simulink model "gdnn_lm_rtrl"  (R2023a)
settings: Solver=ode5  StartTime=0.0  StopTime=train_length  FixedStep=T_sim  RelTol=1e-3  EnableMultiTasking=on
values from neighbouring files (symbols this model uses):
  aa = (((m*l)^2)*g)/AA    (= 0.275046740282)    [init_model.m]
  bb = zeros(1, numoflayers)    [ini_gdnn.m]    (also in init_model.m = 0.588785047389)
  bs = zeros(1, numoflayers)    [ini_gdnn.m]
  cc = (b*m*l)/AA    (= 4.42542074273e-05)    [init_model.m]
  D_max = max(max(max(max(idel))),max(max(max(ldel))))    [ini_gdnn.m]
  dd = (m*g*l*(M+m))/AA    (= 6.05102828621)    [init_model.m]
  DI_vec = [DI_vec DI(i,:)]    [ini_gdnn.m]
  DIB_vec = [DIB_vec DIB(i,:)]    [ini_gdnn.m]
  dimax = max(dimax)    [ini_gdnn.m]
  DIS_vec = [DIS_vec DIS(i,:)]    [ini_gdnn.m]
  DL_vec = [DL_vec DL(i,:)]    [ini_gdnn.m]
  DLB_vec = [DLB_vec DLB(i,:)]    [ini_gdnn.m]
  dlmax = max(dlmax)    [ini_gdnn.m]
  DLS_vec = [DLS_vec DLS(i,:)]    [ini_gdnn.m]
  E_LW_U = zeros(1,numoflayers^2)    [ini_gdnn.m]
  ee = (m*l*c)/AA    (= 0.353271042564)    [init_model.m]
  ff = ((M+m)*b)/AA    (= 0.0009735925634)    [init_model.m]
  I = zeros(1,numoflayers*numofinputs)    [ini_gdnn.m]    (also in init_model.m = 0.05833333)
  idelb_vec = 0    [ini_gdnn.m]
  idels_vec = 0    [ini_gdnn.m]
  Lb = zeros(1,numoflayers^2)    [ini_gdnn.m]
  ldelb_vec = 0    [ini_gdnn.m]
  ldels_vec = 0    [ini_gdnn.m]
  Lf = zeros(1,numoflayers^2)    [ini_gdnn.m]
  mm = (I +m*(l^2))/AA    (= 0.9345794403)    [init_model.m]
  net_params = [Q, mue, theta, T, L, D_max, numoflayers, numofinputs, max(S), sum(R), S_out, S_target, print_weights, min_weights, prune_interval, train_length, prune_maxerr_OBS, prune_maxerr_exact]    [ini_gdnn.m]
  nn = (m*l)/AA    (= 0.56074768661)    [init_model.m]
  oo = (2*l*(M+m))/AA    (= 12.3364491054)    [init_model.m]
  Q = 500    [ini_gdnn.m]
  T = 0.01    [ini_gdnn.m]
  thetastart = pi    (= 3.14159265359)    [init_model.m]
  thetastartdelta = 10*(pi/180)    (= 0.174532925199)    [init_model.m]
  U = U_target    [ini_gdnn.m]
  U_out = zeros(1, numoflayers)    [ini_gdnn.m]
  U_target = zeros(1, numoflayers)    [ini_gdnn.m]
  W_alpha_ini = ones(1,L)    [ini_gdnn.m]
  W_ini = rand(1,L) - 0.5    [ini_gdnn.m]
  X = zeros(1,numoflayers)    [ini_gdnn.m]
  xstart = 0.0    (= 0)    [init_model.m]
  xstartdelta = 0.0    (= 0)    [init_model.m]
undefined symbols (not defined in the file or in its folder): idel_vec, ldel_vec, R, S
libraries: simulink x2, slpidlib x1
settings Model: Creator=endisch  LastModifiedBy=Wolfgang
settings SolverCC: AlgebraicLoopSolver=TrustRegion
settings DataIOCC: LimitDataPoints=on  SaveFormat=Array  SignalLoggingSaveFormat=ModelDataLogs  ReturnWorkspaceOutputs=off
settings OptimizationCC: InitFltsAndDblsToZero=on  LifeSpan=inf
settings DebuggingCC: SaveWithParameterizedLinksMsg=none  UnderspecifiedInitializationDetection=Classic  MergeDetectMultiDrivingBlocksExec=none  SignalResolutionControl=TryResolveAllWithWarning  SolverPrmCheckMsg=warning  MultiTaskDSMMsg=warning  MultiTaskCondExecSysMsg=none  FcnCallInpInsideContextMsg=warning  UnconnectedInputMsg=warning  UnconnectedOutputMsg=warning  UnconnectedLineMsg=warning  StateNameClashWarn=warning  SFUnexpectedBacktrackingDiag=warning  SFNoUnconditionalDefaultTransitionDiag=warning  SFExecutionAtInitializationDiag=none  ArithmeticOperatorsInVariantConditions=warning
settings HardwareCC: ProdBitPerPointer=32  ProdBitPerSizeT=32  ProdBitPerPtrDiffT=32  ProdLargestAtomicFloat=None  ProdIntDivRoundTo=Undefined  ProdEndianess=Unspecified  ProdWordSize=32  ProdHWDeviceType=32-bit Generic
settings ModelReferenceCC: EnableRefExpFcnMdlSchedulingChecks=on  PropagateSignalLabelsOutOfModel=off
settings SFSimCC: SimUseLocalCustomCode=off  CustomCodeUndefinedFunction=UseInterfaceOnly
settings RTWCC: RTWUseLocalCustomCode=off
settings CodeAppCC: StateflowObjectComments=on
settings GRTTargetCC: TargetFcnLib=ansi_tfl_tmw.mat  TargetLangStandard=C89/C90 (ANSI)  CombineOutputUpdateFcns=off  GRTInterface=on
settings ConfigComp: CovMetricSettings=dw  CovSaveCumulativeToWorkspaceVar=on  CovSaveSingleToWorkspaceVar=on  CovExternalEMLEnable=off

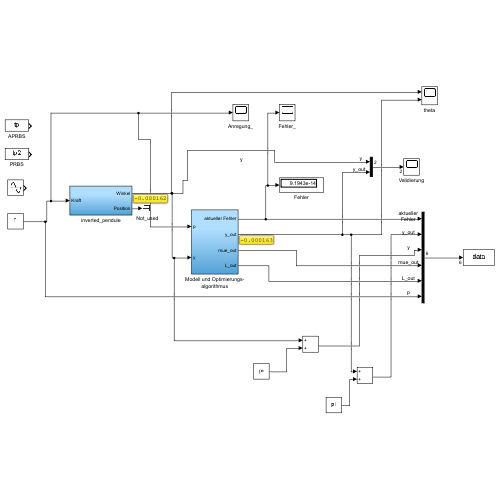
[thumbnail: Simulink's stored preview of the top-level diagram]
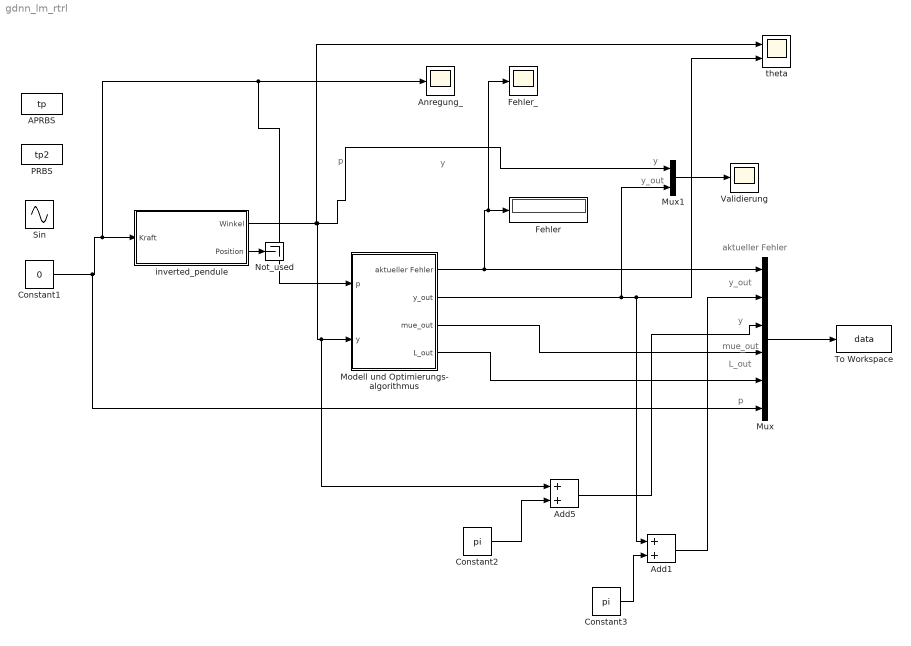
== system gdnn_lm_rtrl ==
  note: y_out
  note: y
  note: y
  note: p
  note: aktueller
      | Fehler
  note: y_out
  note: y
  note: mue_out
  note: L_out
  note: p
  APRBS : FromWorkspace  VariableName=tp  SampleTime=T  Interpolate=off  ZeroCross=off  OutputAfterFinalValue=Cyclic repetition
  Add1 : Sum
  Add5 : Sum
  Anregung_ : Scope
  Constant1 : Constant  Value=0
  Constant2 : Constant  Value=pi
  Constant3 : Constant  Value=pi
  Fehler : Display
      settings: Format=short_e
  "Fehler_ " : Scope
  Modell und Optimierungs- algorithmus : Subsystem
  Mux : Mux  Inputs=6
  Mux1 : Mux  Inputs=2
  Not_used : Terminator
  PRBS : FromWorkspace  VariableName=tp2  SampleTime=T  Interpolate=off  ZeroCross=off  OutputAfterFinalValue=Cyclic repetition
  Sin : Sin  Frequency=0.1  SampleTime=0
  To Workspace : ToWorkspace  VariableName=data  SaveFormat=Structure With Time  SampleTime=-1
  Validierung : Scope
  "inverted_pendule " : Subsystem  AncestorBlock=nichtlinearitaeten/Narendra Example 4
      settings: LibrarySourceBlock=|
      | nichtlinearitaeten/Narendra
      | Example 4
  theta : Scope  NumInputPorts=2
  wires:
  Mux/1 -> To Workspace/1
  "inverted_pendule "/1(Winkel) -> theta/1, Mux1/1, Add5/1, Modell und Optimierungs- algorithmus/2(y)
  Modell und Optimierungs- algorithmus/1(aktueller Fehler) -> "Fehler_ "/1, Fehler/1, Mux/1
  Modell und Optimierungs- algorithmus/3(mue_out) -> Mux/4
  Modell und Optimierungs- algorithmus/4(L_out) -> Mux/5
  Mux1/1 -> Validierung/1
  Modell und Optimierungs- algorithmus/2(y_out) -> Mux1/2, Add1/1, theta/2
  "inverted_pendule "/2(Position) -> Not_used/1
  Add5/1 -> Mux/3
  Constant2/1 -> Add5/2
  Add1/1 -> Mux/2
  Constant3/1 -> Add1/2
  Constant1/1 -> Mux/6, Modell und Optimierungs- algorithmus/1(p), Anregung_/1, "inverted_pendule "/1(Kraft)

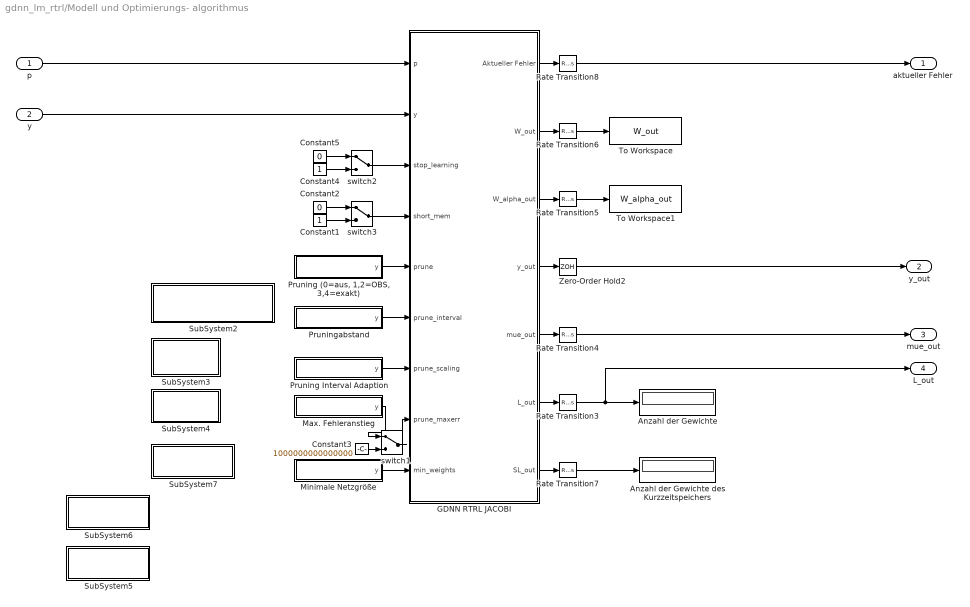
== system gdnn_lm_rtrl/Modell und Optimierungs- algorithmus ==
  p : Inport
  y : Inport  Port=2
  Anzahl der Gewichte : Display
  Anzahl der Gewichte des Kurzzeitspeichers : Display
  Constant1 : Constant
  Constant2 : Constant  Value=0
  Constant3 : Constant  Value=1000000000000000
  Constant4 : Constant
  Constant5 : Constant  Value=0
  GDNN RTRL JACOBI : Subsystem  TreatAsAtomicUnit=on  SystemSampleTime=T
  Max. Fehleranstieg : Subsystem  TreatAsAtomicUnit=on  SystemSampleTime=T  mask(Max. Error After Pruning-Step){number=10}
      mask prompts: number "Max. zulässig ist alter Fehler mal:"
      mask help: 0: Slider inaktiv, Wert wird aus der Ini-Datei (ini_gdnn.m) genommen
      mask Display: disp(sprintf('Fehleranstieg: %.1f',number));
  Minimale Netzgröße : Subsystem  TreatAsAtomicUnit=on  SystemSampleTime=T  mask(Minimum Number of Weights){number=1}
      mask prompts: number "Minimale Anzahl an Gewichte:"
      mask help: 0: Slider inaktiv, Wert wird aus der Ini-Datei (ini_gdnn.m) genommen
      mask Display: disp(sprintf('Gewichte: %i',number));
  "Pruning (0=aus, 1,2=OBS, 3,4=exakt)" : Subsystem  TreatAsAtomicUnit=on  SystemSampleTime=T  mask(Pruning Algorithms){number=0}
      mask prompts: number "Pruningverfahren:"
      mask help:
      | 0: aus
      | 1: OBS
      | 2: OBS, Berücksichtigung der Verzögerungsordnung
      | 3: exaktes Pruning
      | 4: exaktes Pruning, Berücksichtigung der Verzögerungsordnung
      mask TypeOptions number: 0 | 1 | 2 | 3 | 4
      mask Display: disp(sprintf('pruning %i',number-1));
  Pruning Interval Adaption : Subsystem  TreatAsAtomicUnit=on  SystemSampleTime=T  mask(Pruning Interval adaption){number=1}
      mask prompts: number "Skalierungsfaktor"
      mask help: 1.0: Pruning Interval wird nicht angepasst, Pruning Interval ist konstant
      mask Display: disp(sprintf('Scaling: %.1f',number));
  Pruningabstand : Subsystem  TreatAsAtomicUnit=on  SystemSampleTime=T  mask(Pruning Interval){number=100}
      mask prompts: number "Intervall (Abstand zweier Pruningschritte):"
      mask help: 0: Slider inaktiv, Wert wird aus der Ini-Datei (ini_gdnn.m) genommen
      mask Display: disp(sprintf('Intervall: %i',number));
  Rate Transition{3..8} (6 alike) : RateTransition  OutPortSampleTime=T
  SubSystem2 : Subsystem
      settings: OpenFcn=edit ini_gdnn.m gdnn_jacobi_rtrl.c forward_step.c get_jacobi_rtrl.c mem_alloc.c mem_free.c pruning_OBS.c w_conv.c transfer.c m_inv.c shift.c print_weights.c definitions.h;
      mask Display: disp('Load source files into editor\n(Double-Click)')
  SubSystem3 : Subsystem
      settings: OpenFcn="mex -v gdnn_jacobi_rtrl.c forward_step.c  get_jacobi_rtrl.c w_conv.c shift.c transfer.c m_inv.c pruning1_4.c mem_alloc.c mem_free.c print_weights.c"
      mask Display: disp('Mex files\n(Double-Click)')
  SubSystem4 : Subsystem
      settings: OpenFcn=clc
      mask Display: disp('Clear screen\n(Double-Click)')
  SubSystem5 : Subsystem
      settings: OpenFcn=|
      | net_params2 = net_params;
      | Q2=Q;
      | D_max2=D_max;
      | 
      | 
      | R2 = R;
      | S2 = S;
      | U2 = U;
      | X2 = X;
      | I2 = I;
      | Lf2 = Lf;
      | Lb2 = Lb;
      | E_LW_U2 = E_LW_U;
      | DI_vec2 = DI_vec;
      | DL_vec2 = DL_vec;
      | dimax2 = dimax;
      | dlmax2 = dlmax;
      | U_out2 = U_out;
      | U_target2 = U_target;
      | W_ini2 = W_out;
      | W_alpha_ini2 = W_alpha_out;
      | idel_vec2 = idel_vec;
      | ldel_vec2 = ldel_vec;
      | 
      | DIS_vec2=DIS_vec;
      | 
      | DLS_vec2=DLS_vec;
      | 
      | idels_vec2=idels_vec;
      | 
      | ldels_vec2=ldels_vec;
      | 
      | bs2=bs;
      | 
      | DIB_vec2=DIB_vec;
      | 
      | DLB_vec2=DLB_vec;
      | 
      | idelb_vec2=idelb_vec;
      | 
      | ldelb_vec2=ldelb_vec;
      | 
      | bb2= bb;
      | 
      | if exist('params.mat','file') ~= 0
      | !del params.mat
      | end
      | save params net_params2 Q2 D_max2 R2 S2 U2 X2 I2 Lf2 Lb2 E_LW_U2 DI_vec2 DL_vec2 dimax2 dlmax2 U_out2 U_target2 W_ini2 W_alpha_ini2 idel_vec2 ldel_vec2 DIS_vec2 DLS_vec2 idels_vec2 ldels_vec2 bs2 DIB_vec2 DLB_vec2 idelb_vec2 ldelb_vec2 bb2 ;
      | 
      | !copy params.mat ..\11.04.07Gesamtmodell\params.mat
      mask Display: disp('Create params.mat\n(Double-Click)')
  SubSystem6 : Subsystem
      settings: OpenFcn=save W W_out W_alpha_out;
      mask Display: disp('Save weights\n(Double-Click)')
  SubSystem7 : Subsystem
      settings: OpenFcn=|
      | load W;
      | W_ini=W_out;
      | W_alpha_ini=W_alpha_out;
      mask Display: disp('Load old weights\n(Double-Click)')
  To Workspace : ToWorkspace  VariableName=W_out  SampleTime=T
      settings: MaxDataPoints=1
  To Workspace1 : ToWorkspace  VariableName=W_alpha_out  SampleTime=T
      settings: MaxDataPoints=1
  Zero-Order Hold2 : ZeroOrderHold  SampleTime=T
  switch1 : ManualSwitch
  switch2 : ManualSwitch
  switch3 : ManualSwitch
  aktueller Fehler : Outport  VectorParamsAs1DForOutWhenUnconnected=off
  y_out : Outport  Port=2  VectorParamsAs1DForOutWhenUnconnected=off
  mue_out : Outport  Port=3  VectorParamsAs1DForOutWhenUnconnected=off
  L_out : Outport  Port=4  VectorParamsAs1DForOutWhenUnconnected=off
  wires:
  p/1 -> GDNN RTRL JACOBI/1(p)
  y/1 -> GDNN RTRL JACOBI/2(y)
  Constant4/1 -> switch2/2
  Rate Transition8/1 -> aktueller Fehler/1
  switch3/1 -> GDNN RTRL JACOBI/4(short_mem)
  GDNN RTRL JACOBI/4(y_out) -> Zero-Order Hold2/1
  "Pruning (0=aus, 1,2=OBS, 3,4=exakt)"/1(y) -> GDNN RTRL JACOBI/5(prune)
  Minimale Netzgröße/1(y) -> GDNN RTRL JACOBI/9(min_weights)
  Rate Transition7/1 -> Anzahl der Gewichte des Kurzzeitspeichers/1
  GDNN RTRL JACOBI/1(Aktueller Fehler) -> Rate Transition8/1
  GDNN RTRL JACOBI/6(L_out) -> Rate Transition3/1
  Pruning Interval Adaption/1(y) -> GDNN RTRL JACOBI/7("prune_scaling ")
  GDNN RTRL JACOBI/5(mue_out) -> Rate Transition4/1
  Constant2/1 -> switch3/1
  Rate Transition3/1 -> L_out/1, Anzahl der Gewichte/1
  Rate Transition5/1 -> To Workspace1/1
  Constant3/1 -> switch1/2
  GDNN RTRL JACOBI/3(W_alpha_out) -> Rate Transition5/1
  Rate Transition4/1 -> mue_out/1
  Constant5/1 -> switch2/1
  Constant1/1 -> switch3/2
  Zero-Order Hold2/1 -> y_out/1
  switch1/1 -> GDNN RTRL JACOBI/8(prune_maxerr)
  Rate Transition6/1 -> To Workspace/1
  Pruningabstand/1(y) -> GDNN RTRL JACOBI/6("prune_interval ")
  GDNN RTRL JACOBI/2(W_out) -> Rate Transition6/1
  GDNN RTRL JACOBI/7(SL_out) -> Rate Transition7/1
  Max. Fehleranstieg/1(y) -> switch1/1
  switch2/1 -> GDNN RTRL JACOBI/3(stop_learning)

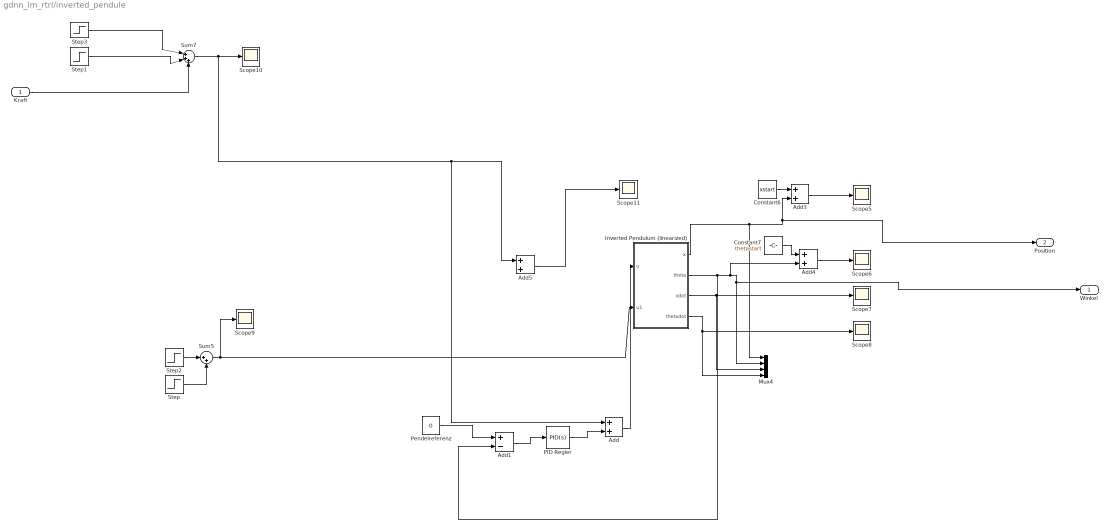
== system gdnn_lm_rtrl/inverted_pendule  ==
  Kraft : Inport
  Add{,3..5} (4 alike) : Sum
  Add1 : Sum  Inputs=+-
  Constant6 : Constant  Value=xstart
  Constant7 : Constant  Value=thetastart
  Inverted Pendulum (linearized) : Subsystem
  Mux4 : Mux
  PID Regler : slpidlib/PID Controller  Controller=PID  Form=Parallel  TimeDomain=Continuous-time  UseExternalTs=off  SampleTime=-1  IntegratorMethod=Forward Euler  FilterMethod=Forward Euler  ControllerParametersSource=internal  P=100  I=1  UseKiTs=off  D=20  N=100  UseFilter=on  TunerSelectOption=Transfer Function Based (PID Tuner App)  InitialConditionSource=internal  InitialConditionForIntegrator=0  InitialConditionForFilter=0  DifferentiatorICPrevScaledInput=0  ExternalReset=none  TrackingMode=off  Kt=1  LimitOutput=off  SatLimitsSource=internal  UpperSaturationLimit=inf  LowerSaturationLimit=-inf  LinearizeAsGain=on  AntiWindupMode=none  Kb=1  LimitIntegrator=off  UpperIntegratorSaturationLimit=inf  LowerIntegratorSaturationLimit=-inf  POutMin=[]  POutMax=[]  IOutMin=[]  IOutMax=[]  DOutMin=[]  DOutMax=[]  NOutMin=[]  NOutMax=[]  SumOutMin=[]  SumOutMax=[]  SaturationOutMin=[]  SaturationOutMax=[]  PParamMin=[]  PParamMax=[]  IParamMin=[]  IParamMax=[]  DParamMin=[]  DParamMax=[]  NParamMin=[]  NParamMax=[]  KbParamMin=[]  KbParamMax=[]  KtParamMin=[]  KtParamMax=[]  KbOutMin=[]  KbOutMax=[]  KtOutMin=[]  KtOutMax=[]  IntegratorOutMin=[]  IntegratorOutMax=[]  FilterOutMin=[]  FilterOutMax=[]  SumI1OutMin=[]  SumI1OutMax=[]  SumI2OutMin=[]  SumI2OutMax=[]  SumI3OutMin=[]  SumI3OutMax=[]  SumI4OutMin=[]  SumI4OutMax=[]  SumDOutMin=[]  SumDOutMax=[]  DifferentiatorOutMin=[]  DifferentiatorOutMax=[]  FilterDiffOutCoefMin=[]  FilterDiffOutCoefMax=[]  ReciprocalOutMin=[]  ReciprocalOutMax=[]  SumDenOutMin=[]  SumDenOutMax=[]  SumNumOutMin=[]  SumNumOutMax=[]  DivideOutMin=[]  DivideOutMax=[]  UdiffTsProdOutMin=[]  UdiffTsProdOutMax=[]  NTsProdOutMin=[]  NTsProdOutMax=[]  UintegralTsProdOutMin=[]  UintegralTsProdOutMax=[]  UngainTsProdOutMin=[]  UngainTsProdOutMax=[]  ClampingZeroOutDataTypeStr=Inherit: Inherit via back propagation  ClampingZeroOutMin=[]  ClampingZeroOutMax=[]  FilterDenConstantOutDataTypeStr=Inherit: Inherit via back propagation  FilterDenConstantOutMin=[]  FilterDenConstantOutMax=[]  PCopyOutDataTypeStr=Inherit: Inherit via back propagation  PCopyOutMin=[]  PCopyOutMax=[]  NCopyOutDataTypeStr=Inherit: Inherit via back propagation  NCopyOutMin=[]  NCopyOutMax=[]  IntegratorContinuousStateAttributes=''  IntegratorStateMustResolveToSignalObject=off  IntegratorRTWStateStorageClass=Auto  FilterContinuousStateAttributes=''  FilterStateMustResolveToSignalObject=off  FilterRTWStateStorageClass=Auto  ParallelPVariant=InternalParameters  IdealPVariant=Disabled  IVariant=InternalParameters  DVariant=InternalParameters  IntegratorVariant=Continuous  SatVariant=Disabled  AWVariant=Passthrough  PCopyVariant=Disabled  TRVariant=Disabled  FdbkBlocksVariant=Forward  IdealPFdbkVariant=Disabled  SatFdbkVariant=Disabled  DerivativeFilterVariant=ContFilter  NVariant=InternalParameters  NCopyVariant=Disabled  FilterICVariant=InternalICsFilter  IntegratorICVariant=InternalICs  ExternalResetVariant=Disabled  TRSumVariant=Passthrough  SumFdbkVariant=Disabled  SumVariant=Sum_PID  TsampFilterVariant=InternalTs  TsampNgainVariant=Passthrough  TsampIntegralVariant=Disabled_SignalSpec  ExternalSaturationOutDataTypeStr=Inherit: Same as second input
  Pendelreferenz : Constant  Value=0
  Scope{5..11} (7 alike) : Scope
  Step : Step  Time=8.1  After=0  SampleTime=0
  Step1 : Step  Time=5.1  After=0  SampleTime=0
  Step2 : Step  Time=8  After=0  SampleTime=0
  Step3 : Step  Time=5  After=0  SampleTime=0
  Sum5 : Sum  Inputs=|++
  Sum7 : Sum  Inputs=|+++
  Winkel : Outport  VectorParamsAs1DForOutWhenUnconnected=off
  Position : Outport  Port=2  VectorParamsAs1DForOutWhenUnconnected=off
  wires:
  Kraft/1 -> Sum7/3
  Constant6/1 -> Add3/1
  Step2/1 -> Sum5/1
  Step1/1 -> Sum7/2
  Inverted Pendulum (linearized)/3(xdot) -> Mux4/3, Scope7/1
  Sum7/1 -> Add/1, Add5/1, Scope10/1
  Step3/1 -> Sum7/1
  Step/1 -> Sum5/2
  Inverted Pendulum (linearized)/4(thetadot) -> Mux4/4, Scope8/1
  Sum5/1 -> Inverted Pendulum (linearized)/2(u1), Scope9/1
  Inverted Pendulum (linearized)/1(x) -> Position/1, Add3/2, Mux4/1
  Inverted Pendulum (linearized)/2(theta) -> Add1/2, Add4/2, Winkel/1, Mux4/2
  Constant7/1 -> Add4/1
  Add3/1 -> Scope5/1
  Add5/1 -> Scope11/1
  Add4/1 -> Scope6/1
  Pendelreferenz/1 -> Add1/1
  Add1/1 -> PID Regler/1
  PID Regler/1 -> Add/2
  Add/1 -> Inverted Pendulum (linearized)/1(u)

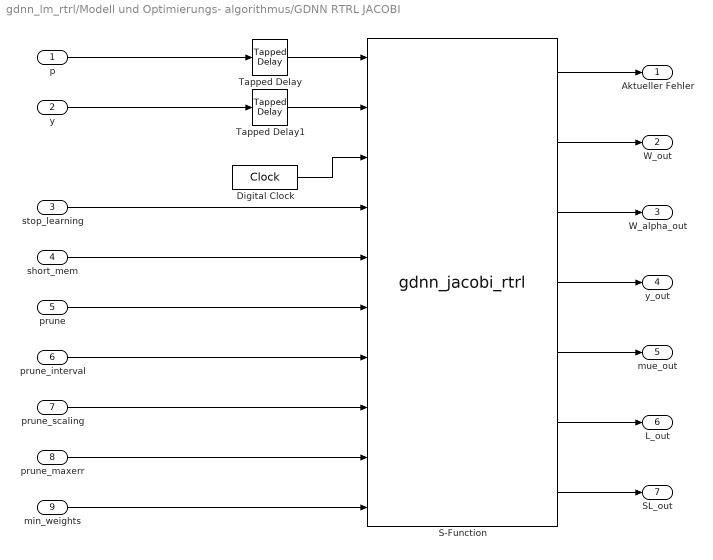
== system gdnn_lm_rtrl/Modell und Optimierungs- algorithmus/GDNN RTRL JACOBI ==
  p : Inport
  y : Inport  Port=2
  stop_learning : Inport  Port=3
  short_mem : Inport  Port=4
  prune : Inport  Port=5
  "prune_interval " : Inport  Port=6
  "prune_scaling " : Inport  Port=7
  prune_maxerr : Inport  Port=8
  min_weights : Inport  Port=9
  Digital Clock : DigitalClock  SampleTime=T
  S-Function : S-Function  FunctionName=gdnn_jacobi_rtrl  Parameters=net_params,R,S,U,X,I,Lf,Lb,E_LW_U,DI_vec,DL_vec,dimax,dlmax,U_out,U_target,W_ini,W_alpha_ini,idel_vec,ldel_vec,DIS_vec,DLS_vec,idels_vec,ldels_vec,bs,DIB_vec,DLB_vec,idelb_vec,ldelb_vec,bb  SFunctionModules=forward_step.c get_jacobi_rtrl.c w_conv.c shift.c transfer.c m_inv.c pruning1_4.c mem_alloc.c mem_free.c  SFunctionDeploymentMode=off  EnableBusSupport=off
  Tapped Delay : simulink/Discrete/Tapped Delay  vinit=0.0  samptime=-1  NumDelays=Q+D_max-1  DelayOrder=Oldest  includeCurrent=on
  Tapped Delay1 : simulink/Discrete/Tapped Delay  vinit=0.0  samptime=-1  NumDelays=Q-1  DelayOrder=Oldest  includeCurrent=on
  Aktueller Fehler : Outport  VectorParamsAs1DForOutWhenUnconnected=off
  W_out : Outport  Port=2  VectorParamsAs1DForOutWhenUnconnected=off
  W_alpha_out : Outport  Port=3  VectorParamsAs1DForOutWhenUnconnected=off
  y_out : Outport  Port=4  VectorParamsAs1DForOutWhenUnconnected=off
  mue_out : Outport  Port=5  VectorParamsAs1DForOutWhenUnconnected=off
  L_out : Outport  Port=6  VectorParamsAs1DForOutWhenUnconnected=off
  SL_out : Outport  Port=7  VectorParamsAs1DForOutWhenUnconnected=off
  wires:
  Digital Clock/1 -> S-Function/3
  S-Function/1 -> Aktueller Fehler/1
  S-Function/2 -> W_out/1
  S-Function/3 -> W_alpha_out/1
  S-Function/4 -> y_out/1
  S-Function/5 -> mue_out/1
  S-Function/6 -> L_out/1
  S-Function/7 -> SL_out/1
  stop_learning/1 -> S-Function/4
  short_mem/1 -> S-Function/5
  prune/1 -> S-Function/6
  "prune_interval "/1 -> S-Function/7
  "prune_scaling "/1 -> S-Function/8
  prune_maxerr/1 -> S-Function/9
  min_weights/1 -> S-Function/10
  y/1 -> Tapped Delay1/1
  Tapped Delay/1 -> S-Function/1
  Tapped Delay1/1 -> S-Function/2
  p/1 -> Tapped Delay/1

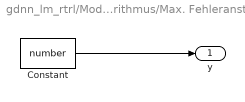
== system gdnn_lm_rtrl/Modell und Optimierungs- algorithmus/Max. Fehleranstieg ==
  Constant : Constant  Value=number
  y : Outport  VectorParamsAs1DForOutWhenUnconnected=off
  wires:
  Constant/1 -> y/1

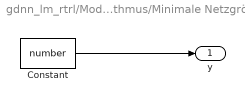
== system gdnn_lm_rtrl/Modell und Optimierungs- algorithmus/Minimale Netzgröße ==
  Constant : Constant  Value=number
  y : Outport  VectorParamsAs1DForOutWhenUnconnected=off
  wires:
  Constant/1 -> y/1

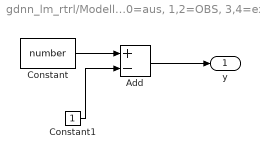
== system gdnn_lm_rtrl/Modell und Optimierungs- algorithmus/Pruning (0=aus, 1,2=OBS, 3,4=exakt) ==
  Add : Sum  Inputs=+-
  Constant : Constant  Value=number
  Constant1 : Constant
  y : Outport  VectorParamsAs1DForOutWhenUnconnected=off
  wires:
  Constant/1 -> Add/1
  Add/1 -> y/1
  Constant1/1 -> Add/2

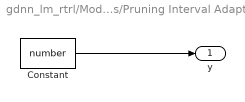
== system gdnn_lm_rtrl/Modell und Optimierungs- algorithmus/Pruning Interval Adaption ==
  Constant : Constant  Value=number
  y : Outport  VectorParamsAs1DForOutWhenUnconnected=off
  wires:
  Constant/1 -> y/1

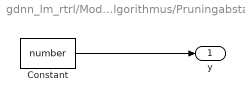
== system gdnn_lm_rtrl/Modell und Optimierungs- algorithmus/Pruningabstand ==
  Constant : Constant  Value=number
  y : Outport  VectorParamsAs1DForOutWhenUnconnected=off
  wires:
  Constant/1 -> y/1

== system gdnn_lm_rtrl/Modell und Optimierungs- algorithmus/SubSystem2 ==

== system gdnn_lm_rtrl/Modell und Optimierungs- algorithmus/SubSystem3 ==

== system gdnn_lm_rtrl/Modell und Optimierungs- algorithmus/SubSystem4 ==

== system gdnn_lm_rtrl/Modell und Optimierungs- algorithmus/SubSystem5 ==

== system gdnn_lm_rtrl/Modell und Optimierungs- algorithmus/SubSystem6 ==

== system gdnn_lm_rtrl/Modell und Optimierungs- algorithmus/SubSystem7 ==

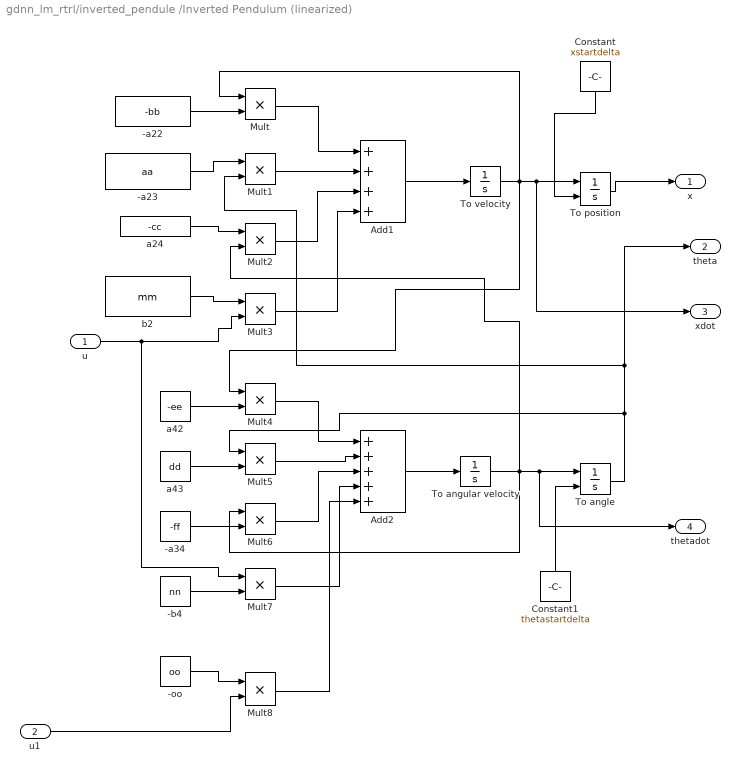
== system gdnn_lm_rtrl/inverted_pendule /Inverted Pendulum (linearized) ==
  u : Inport
  u1 : Inport  Port=2
  -a22 : Constant  Value=-bb
  -a23 : Constant  Value=aa
  -a34 : Constant  Value=-ff
  -b4 : Constant  Value=nn
  -oo : Constant  Value=oo
  Add1 : Sum  Inputs=++++
  Add2 : Sum  Inputs=+++++
  Constant : Constant  Value=xstartdelta
  Constant1 : Constant  Value=thetastartdelta
  Mult{,1..8} (9 alike) : Product  Inputs=**
  To angle : Integrator  InitialConditionSource=external  InitialCondition=1.5
  To angular velocity : Integrator
  To position : Integrator  InitialConditionSource=external  InitialCondition=1
  To velocity : Integrator
  a24 : Constant  Value=-cc
  a42 : Constant  Value=-ee
  a43 : Constant  Value=dd
  b2 : Constant  Value=mm
  x : Outport  VectorParamsAs1DForOutWhenUnconnected=off
  theta : Outport  Port=2  VectorParamsAs1DForOutWhenUnconnected=off
  xdot : Outport  Port=3  VectorParamsAs1DForOutWhenUnconnected=off
  thetadot : Outport  Port=4  VectorParamsAs1DForOutWhenUnconnected=off
  wires:
  -a22/1 -> Mult/2
  Add2/1 -> To angular velocity/1
  -a34/1 -> Mult6/2
  -b4/1 -> Mult7/2
  Mult6/1 -> Add2/3
  Mult3/1 -> Add1/4
  Mult1/1 -> Add1/2
  Add1/1 -> To velocity/1
  b2/1 -> Mult3/1
  To angular velocity/1 -> Mult6/1, Mult2/2, thetadot/1, To angle/1
  -a23/1 -> Mult1/1
  To velocity/1 -> Mult4/1, Mult/1, xdot/1, To position/1
  To angle/1 -> theta/1, Mult1/2, Mult5/1
  Mult7/1 -> Add2/4
  a43/1 -> Mult5/2
  Mult4/1 -> Add2/1
  Mult2/1 -> Add1/3
  u/1 -> Mult7/1, Mult3/2
  a42/1 -> Mult4/2
  Mult/1 -> Add1/1
  Mult5/1 -> Add2/2
  a24/1 -> Mult2/1
  To position/1 -> x/1
  Constant1/1 -> To angle/2
  Constant/1 -> To position/2
  Mult8/1 -> Add2/5
  -oo/1 -> Mult8/1
  u1/1 -> Mult8/2
